simulink model "PODPWM"  (R2013a)
settings: Solver=ode45  StartTime=0.0  StopTime=10.0  RelTol=1e-3
libraries: simulink x20
settings Model: Creator=ASUS  LastModifiedBy=ASUS

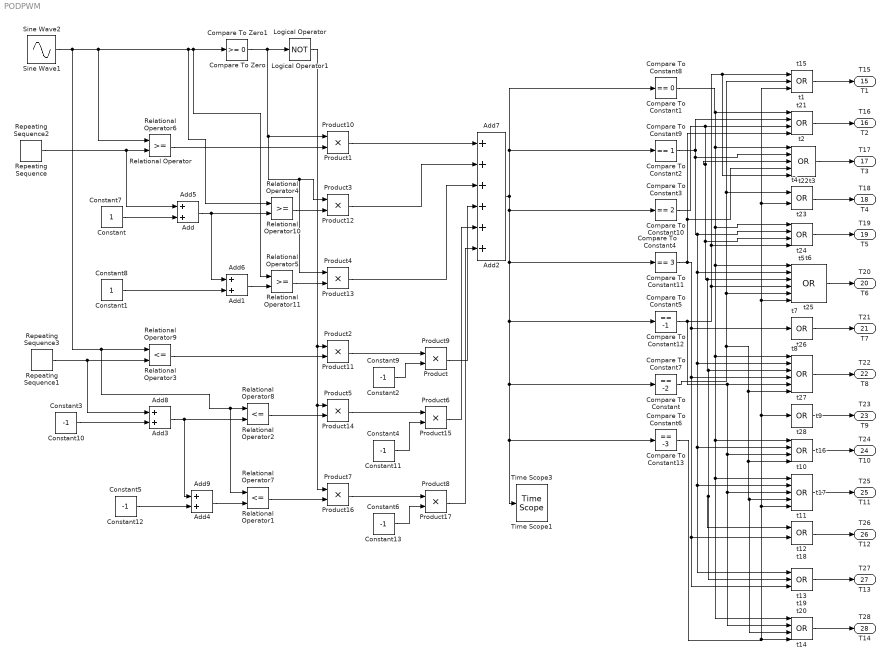
== system PODPWM ==
  Add{,1,3..6,8..9} (8 alike) : Sum
  Add2 : Sum  Inputs=++++++
  Add7 : Sum  Inputs=++++++
  Compare To Constant : simulink/Logic and Bit Operations/Compare To Constant  relop===  const=-2  OutDataTypeStr=boolean
  Compare To Constant1 : simulink/Logic and Bit Operations/Compare To Constant  relop===  const=0  OutDataTypeStr=boolean
  Compare To Constant10 : simulink/Logic and Bit Operations/Compare To Constant  relop===  const=2  OutDataTypeStr=boolean
  Compare To Constant11 : simulink/Logic and Bit Operations/Compare To Constant  relop===  const=3  OutDataTypeStr=boolean
  Compare To Constant12 : simulink/Logic and Bit Operations/Compare To Constant  relop===  const=-1  OutDataTypeStr=boolean
  Compare To Constant13 : simulink/Logic and Bit Operations/Compare To Constant  relop===  const=-3  OutDataTypeStr=boolean
  Compare To Constant2 : simulink/Logic and Bit Operations/Compare To Constant  relop===  const=1  OutDataTypeStr=boolean
  Compare To Constant3 : simulink/Logic and Bit Operations/Compare To Constant  relop===  const=2  OutDataTypeStr=boolean
  Compare To Constant4 : simulink/Logic and Bit Operations/Compare To Constant  relop===  const=3  OutDataTypeStr=boolean
  Compare To Constant5 : simulink/Logic and Bit Operations/Compare To Constant  relop===  const=-1  OutDataTypeStr=boolean
  Compare To Constant6 : simulink/Logic and Bit Operations/Compare To Constant  relop===  const=-3  OutDataTypeStr=boolean
  Compare To Constant7 : simulink/Logic and Bit Operations/Compare To Constant  relop===  const=-2  OutDataTypeStr=boolean
  Compare To Constant8 : simulink/Logic and Bit Operations/Compare To Constant  relop===  const=0  OutDataTypeStr=boolean
  Compare To Constant9 : simulink/Logic and Bit Operations/Compare To Constant  relop===  const=1  OutDataTypeStr=boolean
  Compare To Zero : simulink/Logic and Bit Operations/Compare To Zero  relop=>=  OutDataTypeStr=boolean
  Compare To Zero1 : simulink/Logic and Bit Operations/Compare To Zero  relop=>=  OutDataTypeStr=boolean
  Constant{,1,7..8} (4 alike) : Constant
  Constant{2..6,9..13} (10 alike) : Constant  Value=-1
  Logical Operator : Logic  Operator=NOT  AllPortsSameDT=off  OutDataTypeStr=boolean
  Logical Operator1 : Logic  Operator=NOT  AllPortsSameDT=off  OutDataTypeStr=boolean
  Product{,1..17} (18 alike) : Product
  Relational Operator{,4..6,10..11} (6 alike) : RelationalOperator  OutDataTypeStr=boolean  ZeroCross=off
  Relational Operator{1..3,7..9} (6 alike) : RelationalOperator  Operator=<=  OutDataTypeStr=boolean
  Repeating Sequence : simulink/Sources/Repeating Sequence  rep_seq_t=[0 1/2000 1/1000]  rep_seq_y=[1 0 1]
  Repeating Sequence1 : simulink/Sources/Repeating Sequence  rep_seq_t=[0 1/2000 1/1000]  rep_seq_y=[-1 0 -1]
  Repeating Sequence2 : simulink/Sources/Repeating Sequence  rep_seq_t=[0 1/2000 1/1000]  rep_seq_y=[1 0 1]
  Repeating Sequence3 : simulink/Sources/Repeating Sequence  rep_seq_t=[0 1/2000 1/1000]  rep_seq_y=[-1 0 -1]
  Sine Wave1 : Sin  Amplitude=2.8  Frequency=2*pi*50  SampleTime=0
  Sine Wave2 : Sin  Amplitude=2.8  Frequency=2*pi*50  SampleTime=0
  Time Scope1 : TimeScope  DefaultConfigurationName=spbscopes.TimeScopeBlockCfg
      settings: CopyFcn=scopeextensions.ScopeBlock.callback(gcbh, 'onBlockCopy', gcbh);  DeleteFcn=scopeextensions.ScopeBlock.callback(gcbh, 'onBlockDelete');  PreSaveFcn=scopeextensions.ScopeBlock.callback(gcbh, 'onModelSave');  NameChangeFcn=scopeextensions.ScopeBlock.callback(gcbh, 'onBlockRename');  CloseFcn=scopeextensions.ScopeBlock.callback(gcbh, 'onBlockClose');  PreDeleteFcn=scopeextensions.ScopeBlock.callback(gcbh, 'onBlockPreDelete');
  Time Scope3 : TimeScope  DefaultConfigurationName=spbscopes.TimeScopeBlockCfg
      settings: CopyFcn=scopeextensions.ScopeBlock.callback(gcbh, 'onBlockCopy', gcbh);  DeleteFcn=scopeextensions.ScopeBlock.callback(gcbh, 'onBlockDelete');  PreSaveFcn=scopeextensions.ScopeBlock.callback(gcbh, 'onModelSave');  NameChangeFcn=scopeextensions.ScopeBlock.callback(gcbh, 'onBlockRename');  CloseFcn=scopeextensions.ScopeBlock.callback(gcbh, 'onBlockClose');  PreDeleteFcn=scopeextensions.ScopeBlock.callback(gcbh, 'onBlockPreDelete');
  t{1,13,15,19} (4 alike) : Logic  Operator=OR  Inputs=3  AllPortsSameDT=off  OutDataTypeStr=boolean
  t{2,5,10,14,16,20..21,24} (8 alike) : Logic  Operator=OR  Inputs=4  AllPortsSameDT=off  OutDataTypeStr=boolean
  t{3,11,17,22} (4 alike) : Logic  Operator=OR  Inputs=5  AllPortsSameDT=off  OutDataTypeStr=boolean
  t{4,12,18,23} (4 alike) : Logic  Operator=OR  AllPortsSameDT=off  OutDataTypeStr=boolean
  t{6,8,25,27} (4 alike) : Logic  Operator=OR  Inputs=6  AllPortsSameDT=off  OutDataTypeStr=boolean
  t{7,9,26,28} (4 alike) : Logic  Operator=OR  Inputs=1  AllPortsSameDT=off  OutDataTypeStr=boolean
  T1 : Outport
  T2 : Outport  Port=2
  T3 : Outport  Port=3
  T4 : Outport  Port=4
  T5 : Outport  Port=5
  T6 : Outport  Port=6
  T7 : Outport  Port=7
  T8 : Outport  Port=8
  T9 : Outport  Port=9
  T10 : Outport  Port=10
  T11 : Outport  Port=11
  T12 : Outport  Port=12
  T13 : Outport  Port=13
  T14 : Outport  Port=14
  T15 : Outport  Port=15
  T16 : Outport  Port=16
  T17 : Outport  Port=17
  T18 : Outport  Port=18
  T19 : Outport  Port=19
  T20 : Outport  Port=20
  T21 : Outport  Port=21
  T22 : Outport  Port=22
  T23 : Outport  Port=23
  T24 : Outport  Port=24
  T25 : Outport  Port=25
  T26 : Outport  Port=26
  T27 : Outport  Port=27
  T28 : Outport  Port=28
  wires:
  Sine Wave1/1 -> Relational Operator1/1, Relational Operator2/1, Relational Operator3/1, Relational Operator/1, Relational Operator4/1, Relational Operator5/1, Compare To Zero/1
  Compare To Zero/1 -> Product4/1, Product3/1, Product1/1, Logical Operator/1
  Constant/1 -> Add/2
  Relational Operator/1 -> Product1/2
  Add/1 -> Add1/1, Relational Operator4/2
  Relational Operator4/1 -> Product3/2
  Constant1/1 -> Add1/2
  Add1/1 -> Relational Operator5/2
  Relational Operator5/1 -> Product4/2
  Product1/1 -> Add2/1
  Product3/1 -> Add2/2
  Repeating Sequence1/1 -> Add3/1, Relational Operator3/2
  Relational Operator3/1 -> Product2/2
  Logical Operator/1 -> Product7/1, Product5/1, Product2/1
  Constant2/1 -> Product/2
  Product2/1 -> Product/1
  Constant3/1 -> Add3/2
  Add3/1 -> Add4/1, Relational Operator2/2
  Relational Operator2/1 -> Product5/2
  Constant4/1 -> Product6/2
  Product5/1 -> Product6/1
  Constant5/1 -> Add4/2
  Add4/1 -> Relational Operator1/2
  Relational Operator1/1 -> Product7/2
  Product7/1 -> Product8/1
  Constant6/1 -> Product8/2
  Add2/1 -> Compare To Constant2/1, Compare To Constant1/1, Compare To Constant3/1, Compare To Constant4/1, Compare To Constant5/1, Compare To Constant6/1, Time Scope1/1, Compare To Constant/1
  Repeating Sequence/1 -> Add/1, Relational Operator/2
  Product4/1 -> Add2/3
  Product/1 -> Add2/4
  Product6/1 -> Add2/5
  Product8/1 -> Add2/6
  Compare To Constant1/1 -> t5/1, t6/1, t8/1, t10/1, t11/1, t14/1, t3/1, t2/1
  Compare To Constant2/1 -> t2/2, t8/2, t11/2, t13/1, t10/2, t6/2, t5/2, t3/2
  Compare To Constant3/1 -> t13/2, t12/1, t8/3, t6/3, t5/3, t3/3, t2/3
  Compare To Constant4/1 -> t13/3, t12/2, t8/4, t7/1, t3/4, t2/4
  Compare To Constant5/1 -> t14/2, t11/3, t10/3, t8/5, t6/4, t5/4, t3/5, t1/1
  Compare To Constant/1 -> t14/3, t11/4, t10/4, t8/6, t6/5, t1/2, t4/1
  Compare To Constant6/1 -> t14/4, t11/5, t9/1, t6/6, t4/2, t1/3
  t1/1 -> T1/1
  t2/1 -> T2/1
  t3/1 -> T3/1
  t4/1 -> T4/1
  t5/1 -> T5/1
  t6/1 -> T6/1
  t7/1 -> T7/1
  t8/1 -> T8/1
  t9/1 -> T9/1
  t10/1 -> T10/1
  t11/1 -> T11/1
  t12/1 -> T12/1
  t13/1 -> T13/1
  t14/1 -> T14/1
  Sine Wave2/1 -> Relational Operator7/1, Relational Operator8/1, Relational Operator9/1, Relational Operator6/1, Relational Operator10/1, Relational Operator11/1, Compare To Zero1/1
  Compare To Zero1/1 -> Product13/1, Product12/1, Product10/1, Logical Operator1/1
  Constant7/1 -> Add5/2
  Relational Operator6/1 -> Product10/2
  Add5/1 -> Add6/1, Relational Operator10/2
  Relational Operator10/1 -> Product12/2
  Constant8/1 -> Add6/2
  Add6/1 -> Relational Operator11/2
  Relational Operator11/1 -> Product13/2
  Product10/1 -> Add7/1
  Product12/1 -> Add7/2
  Repeating Sequence3/1 -> Add8/1, Relational Operator9/2
  Relational Operator9/1 -> Product11/2
  Logical Operator1/1 -> Product16/1, Product14/1, Product11/1
  Constant9/1 -> Product9/2
  Product11/1 -> Product9/1
  Constant10/1 -> Add8/2
  Add8/1 -> Add9/1, Relational Operator8/2
  Relational Operator8/1 -> Product14/2
  Constant11/1 -> Product15/2
  Product14/1 -> Product15/1
  Constant12/1 -> Add9/2
  Add9/1 -> Relational Operator7/2
  Relational Operator7/1 -> Product16/2
  Product16/1 -> Product17/1
  Constant13/1 -> Product17/2
  Add7/1 -> Compare To Constant9/1, Compare To Constant8/1, Compare To Constant10/1, Compare To Constant11/1, Compare To Constant12/1, Compare To Constant13/1, Time Scope3/1, Compare To Constant7/1
  Repeating Sequence2/1 -> Add5/1, Relational Operator6/2
  Product13/1 -> Add7/3
  Product9/1 -> Add7/4
  Product15/1 -> Add7/5
  Product17/1 -> Add7/6
  Compare To Constant8/1 -> t24/1, t25/1, t27/1, t16/1, t17/1, t20/1, t22/1, t21/1
  Compare To Constant9/1 -> t21/2, t27/2, t17/2, t19/1, t16/2, t25/2, t24/2, t22/2
  Compare To Constant10/1 -> t19/2, t18/1, t27/3, t25/3, t24/3, t22/3, t21/3
  Compare To Constant11/1 -> t19/3, t18/2, t27/4, t26/1, t22/4, t21/4
  Compare To Constant12/1 -> t20/2, t17/3, t16/3, t27/5, t25/4, t24/4, t22/5, t15/1
  Compare To Constant7/1 -> t20/3, t17/4, t16/4, t27/6, t25/5, t15/2, t23/1
  Compare To Constant13/1 -> t20/4, t17/5, t28/1, t25/6, t23/2, t15/3
  t15/1 -> T15/1
  t21/1 -> T16/1
  t22/1 -> T17/1
  t23/1 -> T18/1
  t24/1 -> T19/1
  t25/1 -> T20/1
  t26/1 -> T21/1
  t27/1 -> T22/1
  t28/1 -> T23/1
  t16/1 -> T24/1
  t17/1 -> T25/1
  t18/1 -> T26/1
  t19/1 -> T27/1
  t20/1 -> T28/1
